simulink model "pendulum_sim"  (R2016b)
settings: Solver=ode45  StartTime=0.0  StopTime=P.t_end  RelTol=1e-3  EnableMultiTasking=on
InitFcn:
  | addpath ./..
  | pendulum_param
  | pendulumParamHW8
undefined symbols (not defined in the file): P, pendulum_animation
settings Model: Creator=beard  LastModifiedBy=mclain
settings DataIOCC: LimitDataPoints=on  SaveFormat=Array  SignalLoggingSaveFormat=ModelDataLogs
settings OptimizationCC: ExpressionDepthLimit=2147483647  InitFltsAndDblsToZero=on  LifeSpan=inf
settings DebuggingCC: UnderspecifiedInitializationDetection=Classic  MergeDetectMultiDrivingBlocksExec=none  SolverPrmCheckMsg=warning  FcnCallInpInsideContextMsg=warning  StateNameClashWarn=warning  SFUnexpectedBacktrackingDiag=warning  SFNoUnconditionalDefaultTransitionDiag=warning  SFExecutionAtInitializationDiag=none
settings HardwareCC: ProdBitPerPointer=32  ProdBitPerSizeT=32  ProdBitPerPtrDiffT=32  ProdLargestAtomicFloat=None  ProdIntDivRoundTo=Undefined  ProdEndianess=Unspecified  ProdWordSize=32  ProdHWDeviceType=32-bit Generic
settings ModelReferenceCC: PropagateSignalLabelsOutOfModel=off
settings GRTTargetCC: TargetLangStandard=C89/C90 (ANSI)  GeneratePreprocessorConditionals=Disable all  CombineOutputUpdateFcns=off  GRTInterface=on
settings ConfigComp: CovMetricSettings=dw  CovHtmlReporting=on  CovSaveCumulativeToWorkspaceVar=on  CovSaveSingleToWorkspaceVar=on  CovExternalEMLEnable=off

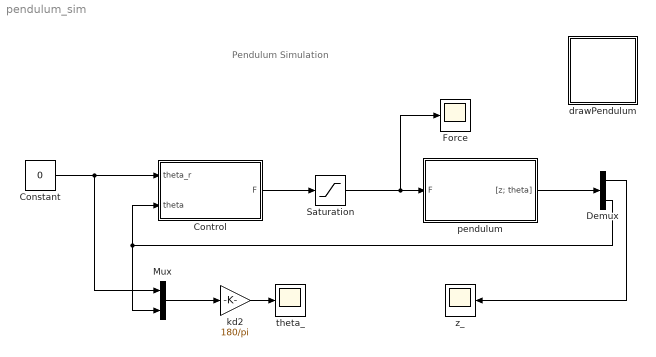
== system pendulum_sim ==
  note: Pendulum Simulation
  Constant : Constant  Value=0
  Control : Subsystem
  Demux : Demux  Outputs=2
  Force : Scope
  Mux : Mux  Inputs=2
  Saturation : Saturate  UpperLimit=P.F_max  LowerLimit=-P.F_max
  drawPendulum : Subsystem
      mask Display: image(imread('tv.jpg'))
  kd2 : Gain  Gain=180/pi
  pendulum : Subsystem
  theta_ : Scope
  z_ : Scope
  wires:
  Control/1(F) -> Saturation/1
  pendulum/1("[z; theta]") -> Demux/1
  Demux/2 -> Mux/2, Control/2(theta)
  Constant/1 -> Mux/1, Control/1(theta_r)
  kd2/1 -> theta_/1
  Mux/1 -> kd2/1
  Demux/1 -> z_/1
  Saturation/1 -> Force/1, pendulum/1(F)

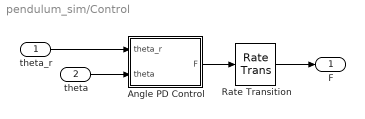
== system pendulum_sim/Control ==
  theta_r : Inport
  theta : Inport  Port=2
  "Angle PD Control " : Subsystem
  Rate Transition : RateTransition  OutPortSampleTime=P.Ts
  F : Outport
  wires:
  theta/1 -> "Angle PD Control "/2(theta)
  theta_r/1 -> "Angle PD Control "/1(theta_r)
  "Angle PD Control "/1(F) -> Rate Transition/1
  Rate Transition/1 -> F/1

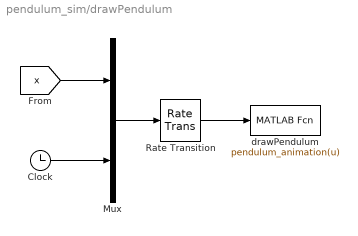
== system pendulum_sim/drawPendulum ==
  Clock : Clock
  Mux : Mux  Inputs=2
  Rate Transition : RateTransition  OutPortSampleTime=P.t_plot
  drawPendulum : MATLABFcn  MATLABFcn=pendulum_animation(u)  OutputDimensions=0
  wires:
  Mux/1 -> Rate Transition/1
  [x] -> Mux/1
  Clock/1 -> Mux/2
  Rate Transition/1 -> drawPendulum/1

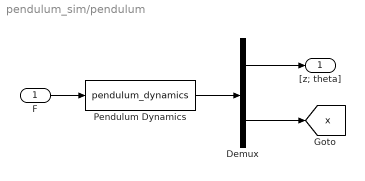
== system pendulum_sim/pendulum ==
  F : Inport
  Demux : Demux  Outputs=[2;4]
  Pendulum Dynamics : S-Function  FunctionName=pendulum_dynamics  Parameters=P  SFunctionDeploymentMode=off  EnableBusSupport=off
  "[z; theta]" : Outport
  tag scope: x=global
  wires:
  F/1 -> Pendulum Dynamics/1
  Pendulum Dynamics/1 -> Demux/1
  Demux/1 -> "[z; theta]"/1
  Demux/2 -> [x]

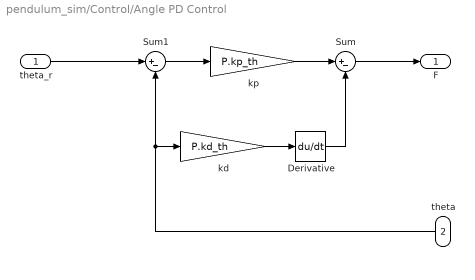
== system pendulum_sim/Control/Angle PD Control  ==
  theta_r : Inport
  theta : Inport  Port=2
  Derivative : Derivative  CoefficientInTFapproximation=P.sigma
  Sum : Sum  Inputs=|+-
  Sum1 : Sum  Inputs=|+-
  kd : Gain  Gain=P.kd_th
  kp : Gain  Gain=P.kp_th
  F : Outport
  wires:
  theta_r/1 -> Sum1/1
  Sum/1 -> F/1
  theta/1 -> kd/1, Sum1/2
  Sum1/1 -> kp/1
  kd/1 -> Derivative/1
  kp/1 -> Sum/1
  Derivative/1 -> Sum/2
